simulink model "MultiMicrogrid"  (R2022b)
settings: Solver=ode45  StartTime=0.0  StopTime=1000  RelTol=1e-3  AbsTol=1e-5
values from neighbouring files (symbols this model uses):
  a_hidden_weights1 = zeros(n,h)    [Weights.m]
  a_hidden_weights2 = zeros(n,h)    [Weights.m]
  a_hidden_weights3 = zeros(n,h)    [Weights.m]
  a_input_weights1 = zeros(h,m)    [Weights.m]
  a_input_weights2 = zeros(h,m)    [Weights.m]
  a_input_weights3 = zeros(h,m)    [Weights.m]
  c_hidden_weights11 = zeros(100,1000)    [Training.m]
  c_hidden_weights12 = -1+(1+1)*rand(1,100,'single')    [Training.m]
  c_hidden_weights21 = zeros(100,1000)    [Training.m]
  c_hidden_weights22 = -1+(1+1)*rand(1,100,'single')    [Training.m]
  c_hidden_weights31 = zeros(100,1000)    [Training.m]
  c_hidden_weights32 = -1+(1+1)*rand(1,100,'single')    [Training.m]
  c_hidden_weights_a1 = -1+(1+1)*rand(1,100,'single')    [Training.m]
  c_hidden_weights_a2 = -1+(1+1)*rand(1,100,'single')    [Training.m]
  c_hidden_weights_a3 = -1+(1+1)*rand(1,100,'single')    [Training.m]
  c_input_weights1 = zeros(1000,m)    [Training.m]
  c_input_weights2 = zeros(1000,m)    [Training.m]
  c_input_weights3 = zeros(1000,m)    [Training.m]
  c_input_weights_a1 = zeros(100,n)    [Training.m]
  c_input_weights_a2 = zeros(100,n)    [Training.m]
  c_input_weights_a3 = zeros(100,n)    [Training.m]
libraries: simulink x27, fuzblock x3, mpclib x3, slpidlib x3
(part 1 of 2)
settings Model: Creator=Vjatšeslav Škiparev  LastModifiedBy=Vjatšeslav Škiparev
settings DataIOCC: SaveState=on  StateSaveName=xout2  TimeSaveName=time  LoggingIntervals=[0, 1000]
settings DebuggingCC: UnconnectedInputMsg=warning  UnconnectedOutputMsg=warning  UnconnectedLineMsg=warning
settings HardwareCC: ProdBitPerLong=64  ProdHWDeviceType=Intel->x86-64 (Linux 64)
settings ModelReferenceCC: EnableRefExpFcnMdlSchedulingChecks=on
settings RTWCC: DLArmComputeVersion=19.05

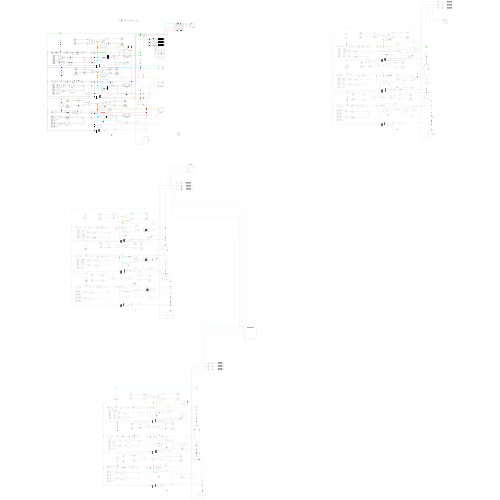
[thumbnail: Simulink's stored preview of the top-level diagram]
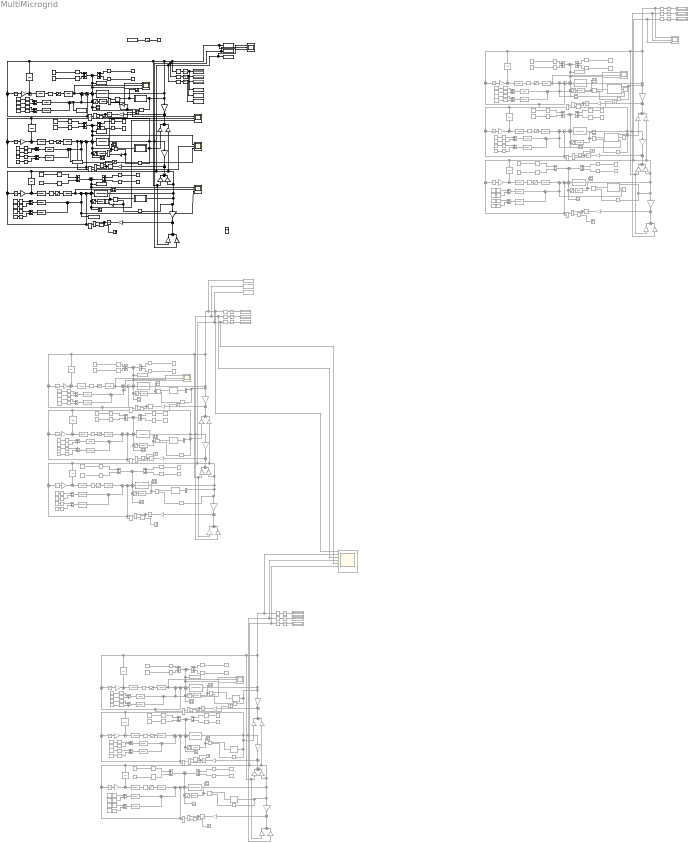
== system MultiMicrogrid ==
  Abs : Abs  SaturateOnIntegerOverflow=off
  Abs1 : Abs  SaturateOnIntegerOverflow=off
  Abs{3..11} (9 alike) : Abs  Commented=on  SaturateOnIntegerOverflow=off
  Abs2 : Abs  SaturateOnIntegerOverflow=off
  Agent 1 : Subsystem
  Agent 2 : Subsystem
  Agent 3 : Subsystem
  Constant : Constant  Value=0.1
  Constant1 : Constant  Value=-0.1
  Constant2 : Constant  SampleTime=1
  Constant3 : Constant  Commented=on  Value=0
  Constant4 : Constant  Commented=on  Value=0
  Constant5 : Constant  Commented=on  Value=0
  Deadband : DeadZone  LowerValue=-0.12  UpperValue=0.12
  Derivative1 : Derivative
  Derivative{4..12} (9 alike) : Derivative  Commented=on
  Derivative2 : Derivative
  Derivative3 : Derivative
  Display : Display
  Display1 : Display
  Display{3..11} (9 alike) : Display  Commented=on
  Display2 : Display
  First Order Hold{1..24} (24 alike) : FirstOrderHold  ErrorTolerance=inf
  First Order Hold{25..96} (72 alike) : FirstOrderHold  Commented=on  ErrorTolerance=inf
  Frequency : Scope  Commented=on  NumInputPorts=8
  Fuzzy Logic Controller1 : fuzblock/Fuzzy Logic  Controller  Commented=on  FIS='test.fis'  OutputSampleNumber=101  DataType=double  FuzzifiedInputs=off  RuleFiringStrengths=off  RuleOutputs=off  AggregatedOutputs=off  SimulateUsing=Interpreted execution  OutOfRangeInputValueMessage=warning  NoRuleFiredMessage=warning  EmptyOutputFuzzySetMessage=warning
  Fuzzy Logic Controller2 : fuzblock/Fuzzy Logic  Controller  Commented=on  FIS='test.fis'  OutputSampleNumber=101  DataType=double  FuzzifiedInputs=off  RuleFiringStrengths=off  RuleOutputs=off  AggregatedOutputs=off  SimulateUsing=Interpreted execution  OutOfRangeInputValueMessage=warning  NoRuleFiredMessage=warning  EmptyOutputFuzzySetMessage=warning
  Fuzzy Logic Controller3 : fuzblock/Fuzzy Logic  Controller  Commented=on  FIS='test.fis'  OutputSampleNumber=101  DataType=double  FuzzifiedInputs=off  RuleFiringStrengths=off  RuleOutputs=off  AggregatedOutputs=off  SimulateUsing=Interpreted execution  OutOfRangeInputValueMessage=warning  NoRuleFiredMessage=warning  EmptyOutputFuzzySetMessage=warning
  GRC : DeadZone  LowerValue=-0.12  UpperValue=0.12
  GRC{1,3..10} (9 alike) : DeadZone  Commented=on  LowerValue=-0.12  UpperValue=0.12
  GRC11 : Saturate  UpperLimit=0.4  LowerLimit=0
  GRC2 : DeadZone  LowerValue=-0.12  UpperValue=0.12
  Gain : Gain  Gain=0.25
  Gain1 : Gain  Gain=0.2
  Gain10 : Gain  Gain=3.14*2
  Gain11 : Gain  Gain=3.14*2
  Gain12 : Gain  Gain=0.2+0.25
  Gain13 : Gain  Gain=0.2+0.12
  Gain14 : Gain  Gain=0.25+0.25
  Gain15 : Gain  Gain=-0.6
  Gain16 : Gain  Gain=-0.6
  Gain17 : Gain  Gain=-0.6
  Gain{18,25,31,33,43,45,49,60,62} (9 alike) : Gain  Commented=on  Gain=0.25
  Gain{19,26,32,44,50,61} (6 alike) : Gain  Commented=on  Gain=0.2
  Gain2 : Gain  Gain=-0.40
  Gain{20..21,27,35..36,47,51,53,64} (9 alike) : Gain  Commented=on  Gain=3.14*2
  Gain22 : Gain  Commented=on  Gain=0.2+0.25
  Gain23 : Gain  Commented=on  Gain=0.2+0.12
  Gain24 : Gain  Commented=on  Gain=0.25+0.25
  Gain28 : Gain  Commented=on  Gain=-0.40
  Gain29 : Gain  Commented=on  Gain=-0.25
  Gain3 : Gain  Gain=-0.25
  Gain30 : Gain  Commented=on  Gain=0.12
  Gain34 : Gain  Commented=on  Gain=-0.35
  Gain37 : Gain  Commented=on  Gain=0.2+0.25
  Gain38 : Gain  Commented=on  Gain=0.2+0.12
  Gain39 : Gain  Commented=on  Gain=0.25+0.25
  Gain4 : Gain  Gain=0.12
  Gain40 : Gain  Commented=on  Gain=-0.40
  Gain41 : Gain  Commented=on  Gain=-0.25
  Gain42 : Gain  Commented=on  Gain=0.12
  Gain46 : Gain  Commented=on  Gain=-0.35
  Gain5 : Gain  Gain=0.25
  Gain54 : Gain  Commented=on  Gain=0.2+0.25
  Gain55 : Gain  Commented=on  Gain=0.2+0.12
  Gain56 : Gain  Commented=on  Gain=0.25+0.25
  Gain57 : Gain  Commented=on  Gain=-0.40
  Gain58 : Gain  Commented=on  Gain=-0.25
  Gain59 : Gain  Commented=on  Gain=0.12
  Gain6 : Gain  Gain=0.2
  Gain63 : Gain  Commented=on  Gain=-0.35
  Gain7 : Gain  Gain=0.25
  Gain8 : Gain  Gain=-0.35
  Gain9 : Gain  Gain=3.14*2
  Industrial Loads1 : UniformRandomNumber  Minimum=-0.01  Maximum=0.01  SampleTime=1
  Industrial Loads{9..10,13,18..19,24} (6 alike) : UniformRandomNumber  Commented=on  Minimum=-0.03  Maximum=0.03  SampleTime=5
  Industrial Loads{11..12,14..15,20..21} (6 alike) : UniformRandomNumber  Commented=on  Minimum=-0.01  Maximum=0.01  SampleTime=2
  Industrial Loads16 : UniformRandomNumber  Commented=on  Minimum=-0.01  Maximum=0.01  SampleTime=1
  Industrial Loads17 : UniformRandomNumber  Commented=on  Minimum=-0.05  Maximum=0.05  SampleTime=2
  Industrial Loads2 : UniformRandomNumber  Minimum=-0.05  Maximum=0.05  SampleTime=2
  Industrial Loads22 : UniformRandomNumber  Commented=on  Minimum=-0.01  Maximum=0.01  SampleTime=1
  Industrial Loads23 : UniformRandomNumber  Commented=on  Minimum=-0.05  Maximum=0.05  SampleTime=2
  Industrial Loads3 : UniformRandomNumber  Minimum=-0.03  Maximum=0.03  SampleTime=5
  Industrial Loads4 : UniformRandomNumber  Minimum=-0.03  Maximum=0.03  SampleTime=5
  Industrial Loads5 : UniformRandomNumber  Minimum=-0.01  Maximum=0.01  SampleTime=2
  Industrial Loads6 : UniformRandomNumber  Minimum=-0.01  Maximum=0.01  SampleTime=2
  Industrial Loads7 : UniformRandomNumber  Commented=on  Minimum=-0.01  Maximum=0.01  SampleTime=1
  Industrial Loads8 : UniformRandomNumber  Commented=on  Minimum=-0.05  Maximum=0.05  SampleTime=2
  Integrator{,1..9} (10 alike) : Integrator
  Integrator{10..36} (27 alike) : Integrator  Commented=on
  Limiter1 : Saturate  Commented=on  UpperLimit=0.4  LowerLimit=0
  Limiter10 : Saturate  Commented=on  LowerLimit=0
  Limiter11 : Saturate  Commented=on  UpperLimit=0.3  LowerLimit=0
  Limiter2 : Saturate  LowerLimit=0
  Limiter3 : Saturate  UpperLimit=0.3  LowerLimit=0
  Limiter4 : Saturate  Commented=on  UpperLimit=0.4  LowerLimit=0
  Limiter5 : Saturate  Commented=on  LowerLimit=0
  Limiter6 : Saturate  Commented=on  UpperLimit=0.3  LowerLimit=0
  Limiter7 : Saturate  Commented=on  LowerLimit=0
  Limiter8 : Saturate  Commented=on  UpperLimit=0.3  LowerLimit=0
  Limiter9 : Saturate  Commented=on  UpperLimit=0.4  LowerLimit=0
  MPC Controller : mpclib/MPC Controller  Commented=on  SCDEnableBlockLinearizationSpecification=on  is_multiple=0  enable_value=0  return_u0=off  updateMPCinCallerWorkspace=on  md_inport=on  mv_inport=off  uref_inport=off  return_cost=off  return_mvseq=off  return_qpstatus=off  return_xseq=off  return_state=off  return_ovseq=off  state_inport=off  umin_inport=off  umax_inport=off  ymin_inport=off  ymax_inport=off  cc_inport=off  ywt_inport=off  uwt_inport=off  duwt_inport=off  rhoeps_inport=off  pm_inport=off  MaximumP=10  HorizonChoice=FixedHorizon  n_ts=1  n_p=10  n_mv=1  n_md=1  n_ud=0  n_mo=1  n_uo=0  BlockDataType=double  SampleTimeInherited=off  switch_inport=off
  MPC Controller1 : mpclib/MPC Controller  Commented=on  SCDEnableBlockLinearizationSpecification=on  is_multiple=0  enable_value=0  return_u0=off  updateMPCinCallerWorkspace=on  md_inport=on  mv_inport=off  uref_inport=off  return_cost=off  return_mvseq=off  return_qpstatus=off  return_xseq=off  return_state=off  return_ovseq=off  state_inport=off  umin_inport=off  umax_inport=off  ymin_inport=off  ymax_inport=off  cc_inport=off  ywt_inport=off  uwt_inport=off  duwt_inport=off  rhoeps_inport=off  pm_inport=off  MaximumP=10  HorizonChoice=FixedHorizon  n_ts=1  n_p=10  n_mv=1  n_md=1  n_ud=0  n_mo=1  n_uo=0  BlockDataType=double  SampleTimeInherited=off  switch_inport=off
  MPC Controller2 : mpclib/MPC Controller  Commented=on  SCDEnableBlockLinearizationSpecification=on  mpcobj=mpc1  is_multiple=0  enable_value=0  return_u0=off  updateMPCinCallerWorkspace=on  md_inport=on  mv_inport=off  uref_inport=off  return_cost=off  return_mvseq=off  return_qpstatus=off  return_xseq=off  return_state=off  return_ovseq=off  state_inport=off  umin_inport=off  umax_inport=off  ymin_inport=off  ymax_inport=off  cc_inport=off  ywt_inport=off  uwt_inport=off  duwt_inport=off  rhoeps_inport=off  pm_inport=off  MaximumP=10  HorizonChoice=FixedHorizon  n_ts=1  n_p=10  n_mv=1  n_md=1  n_ud=0  n_mo=1  n_uo=0  BlockDataType=double  SampleTimeInherited=off  switch_inport=off
  Manual Variant Source{6..11} (6 alike) : simulink/Signal Routing/Manual Variant Source  NumChoices=2  LabelModeActiveChoice=V_2
  Manual Variant Source{2,12..14,16..19,22,24..28} (14 alike) : simulink/Signal Routing/Manual Variant Source  Commented=on  NumChoices=2  LabelModeActiveChoice=V_2
  Manual Variant Source{15,20..21,23} (4 alike) : simulink/Signal Routing/Manual Variant Source  Commented=on  NumChoices=2  LabelModeActiveChoice=V_1
  Manual Variant Source3 : simulink/Signal Routing/Manual Variant Source  NumChoices=2  LabelModeActiveChoice=V_1
  Manual Variant Source4 : simulink/Signal Routing/Manual Variant Source  NumChoices=2  LabelModeActiveChoice=V_1
  Manual Variant Source5 : simulink/Signal Routing/Manual Variant Source  NumChoices=2  LabelModeActiveChoice=V_1
  Mux1 : Mux  Commented=on  Inputs=2
  Mux2 : Mux  Commented=on  Inputs=2
  Mux3 : Mux  Commented=on  Inputs=2
  PID Controller1 : slpidlib/PID Controller  Commented=on  Controller=PID  Form=Parallel  TimeDomain=Continuous-time  UseExternalTs=off  SampleTime=-1  IntegratorMethod=Forward Euler  FilterMethod=Forward Euler  ControllerParametersSource=internal  P=7.5  I=2.5  UseKiTs=off  D=0.75  N=100  UseFilter=on  TunerSelectOption=Transfer Function Based (PID Tuner App)  InitialConditionSource=internal  InitialConditionForIntegrator=0  InitialConditionForFilter=0  DifferentiatorICPrevScaledInput=0  ExternalReset=none  TrackingMode=off  Kt=1  LimitOutput=off  SatLimitsSource=internal  UpperSaturationLimit=inf  LowerSaturationLimit=0  LinearizeAsGain=on  AntiWindupMode=none  Kb=1  LimitIntegrator=off  UpperIntegratorSaturationLimit=inf  LowerIntegratorSaturationLimit=-inf  POutMin=[]  POutMax=[]  IOutMin=[]  IOutMax=[]  DOutMin=[]  DOutMax=[]  NOutMin=[]  NOutMax=[]  SumOutMin=[]  SumOutMax=[]  SaturationOutMin=[]  SaturationOutMax=[]  PParamMin=[]  PParamMax=[]  IParamMin=[]  IParamMax=[]  DParamMin=[]  DParamMax=[]  NParamMin=[]  NParamMax=[]  KbParamMin=[]  KbParamMax=[]  KtParamMin=[]  KtParamMax=[]  KbOutMin=[]  KbOutMax=[]  KtOutMin=[]  KtOutMax=[]  IntegratorOutMin=[]  IntegratorOutMax=[]  FilterOutMin=[]  FilterOutMax=[]  SumI1OutMin=[]  SumI1OutMax=[]  SumI2OutMin=[]  SumI2OutMax=[]  SumI3OutMin=[]  SumI3OutMax=[]  SumI4OutMin=[]  SumI4OutMax=[]  SumDOutMin=[]  SumDOutMax=[]  DifferentiatorOutMin=[]  DifferentiatorOutMax=[]  FilterDiffOutCoefMin=[]  FilterDiffOutCoefMax=[]  ReciprocalOutMin=[]  ReciprocalOutMax=[]  SumDenOutMin=[]  SumDenOutMax=[]  SumNumOutMin=[]  SumNumOutMax=[]  DivideOutMin=[]  DivideOutMax=[]  UdiffTsProdOutMin=[]  UdiffTsProdOutMax=[]  NTsProdOutMin=[]  NTsProdOutMax=[]  UintegralTsProdOutMin=[]  UintegralTsProdOutMax=[]  UngainTsProdOutMin=[]  UngainTsProdOutMax=[]  ClampingZeroOutDataTypeStr=Inherit: Inherit via back propagation  ClampingZeroOutMin=[]  ClampingZeroOutMax=[]  FilterDenConstantOutDataTypeStr=Inherit: Inherit via back propagation  FilterDenConstantOutMin=[]  FilterDenConstantOutMax=[]  PCopyOutDataTypeStr=Inherit: Inherit via back propagation  PCopyOutMin=[]  PCopyOutMax=[]  NCopyOutDataTypeStr=Inherit: Inherit via back propagation  NCopyOutMin=[]  NCopyOutMax=[]  IntegratorContinuousStateAttributes=''  IntegratorStateMustResolveToSignalObject=off  IntegratorRTWStateStorageClass=Auto  FilterContinuousStateAttributes=''  FilterStateMustResolveToSignalObject=off  FilterRTWStateStorageClass=Auto  ParallelPVariant=InternalParameters  IdealPVariant=Disabled  IVariant=InternalParameters  DVariant=InternalParameters  IntegratorVariant=Continuous  SatVariant=Disabled  AWVariant=Passthrough  PCopyVariant=Disabled  TRVariant=Disabled  FdbkBlocksVariant=Forward  IdealPFdbkVariant=Disabled  SatFdbkVariant=Disabled  DerivativeFilterVariant=ContFilter  NVariant=InternalParameters  NCopyVariant=Disabled  FilterICVariant=InternalICsFilter  IntegratorICVariant=InternalICs  ExternalResetVariant=Disabled  TRSumVariant=Passthrough  SumFdbkVariant=Disabled  SumVariant=Sum_PID  TsampFilterVariant=InternalTs  TsampNgainVariant=Passthrough  TsampIntegralVariant=Passthrough  ExternalSaturationOutDataTypeStr=Inherit: Same as second input
  PID Controller2 : slpidlib/PID Controller  Commented=on  Controller=PID  Form=Parallel  TimeDomain=Continuous-time  UseExternalTs=off  SampleTime=-1  IntegratorMethod=Forward Euler  FilterMethod=Forward Euler  ControllerParametersSource=internal  P=4.75  I=1.25  UseKiTs=off  D=0.5  N=100  UseFilter=on  TunerSelectOption=Transfer Function Based (PID Tuner App)  InitialConditionSource=internal  InitialConditionForIntegrator=0  InitialConditionForFilter=0  DifferentiatorICPrevScaledInput=0  ExternalReset=none  TrackingMode=off  Kt=1  LimitOutput=off  SatLimitsSource=internal  UpperSaturationLimit=inf  LowerSaturationLimit=-inf  LinearizeAsGain=on  AntiWindupMode=back-calculation  Kb=1  LimitIntegrator=off  UpperIntegratorSaturationLimit=inf  LowerIntegratorSaturationLimit=-inf  POutMin=[]  POutMax=[]  IOutMin=[]  IOutMax=[]  DOutMin=[]  DOutMax=[]  NOutMin=[]  NOutMax=[]  SumOutMin=[]  SumOutMax=[]  SaturationOutMin=[]  SaturationOutMax=[]  PParamMin=[]  PParamMax=[]  IParamMin=[]  IParamMax=[]  DParamMin=[]  DParamMax=[]  NParamMin=[]  NParamMax=[]  KbParamMin=[]  KbParamMax=[]  KtParamMin=[]  KtParamMax=[]  KbOutMin=[]  KbOutMax=[]  KtOutMin=[]  KtOutMax=[]  IntegratorOutMin=[]  IntegratorOutMax=[]  FilterOutMin=[]  FilterOutMax=[]  SumI1OutMin=[]  SumI1OutMax=[]  SumI2OutMin=[]  SumI2OutMax=[]  SumI3OutMin=[]  SumI3OutMax=[]  SumI4OutMin=[]  SumI4OutMax=[]  SumDOutMin=[]  SumDOutMax=[]  DifferentiatorOutMin=[]  DifferentiatorOutMax=[]  FilterDiffOutCoefMin=[]  FilterDiffOutCoefMax=[]  ReciprocalOutMin=[]  ReciprocalOutMax=[]  SumDenOutMin=[]  SumDenOutMax=[]  SumNumOutMin=[]  SumNumOutMax=[]  DivideOutMin=[]  DivideOutMax=[]  UdiffTsProdOutMin=[]  UdiffTsProdOutMax=[]  NTsProdOutMin=[]  NTsProdOutMax=[]  UintegralTsProdOutMin=[]  UintegralTsProdOutMax=[]  UngainTsProdOutMin=[]  UngainTsProdOutMax=[]  ClampingZeroOutDataTypeStr=Inherit: Inherit via back propagation  ClampingZeroOutMin=[]  ClampingZeroOutMax=[]  FilterDenConstantOutDataTypeStr=Inherit: Inherit via back propagation  FilterDenConstantOutMin=[]  FilterDenConstantOutMax=[]  PCopyOutDataTypeStr=Inherit: Inherit via back propagation  PCopyOutMin=[]  PCopyOutMax=[]  NCopyOutDataTypeStr=Inherit: Inherit via back propagation  NCopyOutMin=[]  NCopyOutMax=[]  IntegratorContinuousStateAttributes=''  IntegratorStateMustResolveToSignalObject=off  IntegratorRTWStateStorageClass=Auto  FilterContinuousStateAttributes=''  FilterStateMustResolveToSignalObject=off  FilterRTWStateStorageClass=Auto  ParallelPVariant=InternalParameters  IdealPVariant=Disabled  IVariant=InternalParameters  DVariant=InternalParameters  IntegratorVariant=Continuous  SatVariant=Disabled  AWVariant=Passthrough  PCopyVariant=Disabled  TRVariant=Disabled  FdbkBlocksVariant=Forward  IdealPFdbkVariant=Disabled  SatFdbkVariant=Disabled  DerivativeFilterVariant=ContFilter  NVariant=InternalParameters  NCopyVariant=Disabled  FilterICVariant=InternalICsFilter  IntegratorICVariant=InternalICs  ExternalResetVariant=Disabled  TRSumVariant=Passthrough  SumFdbkVariant=Disabled  SumVariant=Sum_PID  TsampFilterVariant=InternalTs  TsampNgainVariant=Passthrough  TsampIntegralVariant=Passthrough  ExternalSaturationOutDataTypeStr=Inherit: Same as second input
  PID Controller3 : slpidlib/PID Controller  Commented=on  Controller=PID  Form=Parallel  TimeDomain=Continuous-time  UseExternalTs=off  SampleTime=-1  IntegratorMethod=Forward Euler  FilterMethod=Forward Euler  ControllerParametersSource=internal  P=4.5  I=1.75  UseKiTs=off  D=0.2  N=100  UseFilter=on  TunerSelectOption=Transfer Function Based (PID Tuner App)  InitialConditionSource=internal  InitialConditionForIntegrator=0  InitialConditionForFilter=0  DifferentiatorICPrevScaledInput=0  ExternalReset=none  TrackingMode=off  Kt=1  LimitOutput=off  SatLimitsSource=internal  UpperSaturationLimit=inf  LowerSaturationLimit=0  LinearizeAsGain=on  AntiWindupMode=none  Kb=1  LimitIntegrator=off  UpperIntegratorSaturationLimit=inf  LowerIntegratorSaturationLimit=-inf  POutMin=[]  POutMax=[]  IOutMin=[]  IOutMax=[]  DOutMin=[]  DOutMax=[]  NOutMin=[]  NOutMax=[]  SumOutMin=[]  SumOutMax=[]  SaturationOutMin=[]  SaturationOutMax=[]  PParamMin=[]  PParamMax=[]  IParamMin=[]  IParamMax=[]  DParamMin=[]  DParamMax=[]  NParamMin=[]  NParamMax=[]  KbParamMin=[]  KbParamMax=[]  KtParamMin=[]  KtParamMax=[]  KbOutMin=[]  KbOutMax=[]  KtOutMin=[]  KtOutMax=[]  IntegratorOutMin=[]  IntegratorOutMax=[]  FilterOutMin=[]  FilterOutMax=[]  SumI1OutMin=[]  SumI1OutMax=[]  SumI2OutMin=[]  SumI2OutMax=[]  SumI3OutMin=[]  SumI3OutMax=[]  SumI4OutMin=[]  SumI4OutMax=[]  SumDOutMin=[]  SumDOutMax=[]  DifferentiatorOutMin=[]  DifferentiatorOutMax=[]  FilterDiffOutCoefMin=[]  FilterDiffOutCoefMax=[]  ReciprocalOutMin=[]  ReciprocalOutMax=[]  SumDenOutMin=[]  SumDenOutMax=[]  SumNumOutMin=[]  SumNumOutMax=[]  DivideOutMin=[]  DivideOutMax=[]  UdiffTsProdOutMin=[]  UdiffTsProdOutMax=[]  NTsProdOutMin=[]  NTsProdOutMax=[]  UintegralTsProdOutMin=[]  UintegralTsProdOutMax=[]  UngainTsProdOutMin=[]  UngainTsProdOutMax=[]  ClampingZeroOutDataTypeStr=Inherit: Inherit via back propagation  ClampingZeroOutMin=[]  ClampingZeroOutMax=[]  FilterDenConstantOutDataTypeStr=Inherit: Inherit via back propagation  FilterDenConstantOutMin=[]  FilterDenConstantOutMax=[]  PCopyOutDataTypeStr=Inherit: Inherit via back propagation  PCopyOutMin=[]  PCopyOutMax=[]  NCopyOutDataTypeStr=Inherit: Inherit via back propagation  NCopyOutMin=[]  NCopyOutMax=[]  IntegratorContinuousStateAttributes=''  IntegratorStateMustResolveToSignalObject=off  IntegratorRTWStateStorageClass=Auto  FilterContinuousStateAttributes=''  FilterStateMustResolveToSignalObject=off  FilterRTWStateStorageClass=Auto  ParallelPVariant=InternalParameters  IdealPVariant=Disabled  IVariant=InternalParameters  DVariant=InternalParameters  IntegratorVariant=Continuous  SatVariant=Disabled  AWVariant=Passthrough  PCopyVariant=Disabled  TRVariant=Disabled  FdbkBlocksVariant=Forward  IdealPFdbkVariant=Disabled  SatFdbkVariant=Disabled  DerivativeFilterVariant=ContFilter  NVariant=InternalParameters  NCopyVariant=Disabled  FilterICVariant=InternalICsFilter  IntegratorICVariant=InternalICs  ExternalResetVariant=Disabled  TRSumVariant=Passthrough  SumFdbkVariant=Disabled  SumVariant=Sum_PID  TsampFilterVariant=InternalTs  TsampNgainVariant=Passthrough  TsampIntegralVariant=Passthrough  ExternalSaturationOutDataTypeStr=Inherit: Same as second input
  PowerPlant1 : Scope  NumInputPorts=3
  PowerPlant2 : Scope  NumInputPorts=3
  PowerPlant3 : Scope  NumInputPorts=3
  PowerPlant{4..7} (4 alike) : Scope  Commented=on  NumInputPorts=3
  Product{,1..5} (6 alike) : Product
  Product{6..23} (18 alike) : Product  Commented=on
  Reward1 : ToWorkspace  VariableName=axis  SampleTime=1
      settings: Save2DSignal=2-D array (concatenate along first dimension)
  Saturation : Saturate  UpperLimit=0.25  LowerLimit=-0.25
  Saturation1 : Saturate  UpperLimit=0.1  LowerLimit=-0.1
  Saturation10 : Saturate  Commented=on  UpperLimit=0.1  LowerLimit=-0.1
  Saturation11 : Saturate  Commented=on  UpperLimit=0.2  LowerLimit=-0.2
  Saturation2 : Saturate  UpperLimit=0.2  LowerLimit=-0.2
  Saturation3 : Saturate  Commented=on  UpperLimit=0.25  LowerLimit=-0.25
  Saturation4 : Saturate  Commented=on  UpperLimit=0.1  LowerLimit=-0.1
  Saturation5 : Saturate  Commented=on  UpperLimit=0.2  LowerLimit=-0.2
  Saturation6 : Saturate  Commented=on  UpperLimit=0.25  LowerLimit=-0.25
  Saturation7 : Saturate  Commented=on  UpperLimit=0.1  LowerLimit=-0.1
  Saturation8 : Saturate  Commented=on  UpperLimit=0.2  LowerLimit=-0.2
  Saturation9 : Saturate  Commented=on  UpperLimit=0.25  LowerLimit=-0.25
  Scope{,1..5} (6 alike) : Scope
  Scope{6..23} (18 alike) : Scope  Commented=on
  Solar1 : TransferFcn  Denominator=[1.5 1]
  Solar10 : TransferFcn  Commented=on  Denominator=[1.5 1]
  Solar11 : TransferFcn  Commented=on  Denominator=[1.3 1]
  Solar12 : TransferFcn  Commented=on  Denominator=[1.75 1]
  Solar2 : TransferFcn  Denominator=[1.3 1]
  Solar3 : TransferFcn  Denominator=[1.75 1]
  Solar4 : TransferFcn  Commented=on  Denominator=[1.5 1]
  Solar5 : TransferFcn  Commented=on  Denominator=[1.3 1]
  Solar6 : TransferFcn  Commented=on  Denominator=[1.75 1]
  Solar7 : TransferFcn  Commented=on  Denominator=[1.5 1]
  Solar8 : TransferFcn  Commented=on  Denominator=[1.3 1]
  Solar9 : TransferFcn  Commented=on  Denominator=[1.75 1]
  Step : Step  Time=750  Before=1  After=0  SampleTime=0
  Step1 : Step  Time=250  Before=1  After=0  SampleTime=0
  Step10 : Step  Commented=on  Time=250  Before=1  After=0  SampleTime=0
  Step11 : Step  Commented=on  Time=500  Before=1  After=0  SampleTime=0
  Step2 : Step  Time=500  Before=1  After=0  SampleTime=0
  Step3 : Step  Commented=on  Time=750  Before=1  After=0  SampleTime=0
  Step4 : Step  Commented=on  Time=250  Before=1  After=0  SampleTime=0
  Step5 : Step  Commented=on  Time=500  Before=1  After=0  SampleTime=0
  Step6 : Step  Commented=on  Time=750  Before=1  After=0  SampleTime=0
  Step7 : Step  Commented=on  Time=250  Before=1  After=0  SampleTime=0
  Step8 : Step  Commented=on  Time=500  Before=1  After=0  SampleTime=0
  Step9 : Step  Commented=on  Time=750  Before=1  After=0  SampleTime=0
  Sum : Sum  Inputs=-++
  Sum1 : Sum  Inputs=-++
  Sum{9..11,15..17,24..38} (21 alike) : Sum
  Sum{41..42,46..48,56..61,63..71,77,80..81,85..87,95..100,102..110,116..117,119..127,133,136..137,141..143,151..155} (63 alike) : Sum  Commented=on
  Sum{62,72..73,101,111..112,118,128..129} (9 alike) : Sum  Commented=on  Inputs=-+|
  Sum{74..76,113..115,130..132} (9 alike) : Sum  Commented=on  Inputs=+-
  Sum12 : Sum  Inputs=|+-
  Sum13 : Sum  Inputs=|+-
  Sum{39..40,51,78..79,90,134..135,146} (9 alike) : Sum  Commented=on  Inputs=-++
  Sum{43..45,82..84,138..140} (9 alike) : Sum  Commented=on  Inputs=|+-
  Sum14 : Sum  Inputs=|+-
  Sum{49..50,52..55,88..89,91..94,144..145,147..150} (18 alike) : Sum  Commented=on  Inputs=|++
  Sum{18..23} (6 alike) : Sum  Inputs=|++
  Sum2 : Sum  Inputs=-++
  Sum3 : Sum  Inputs=-+|
  Sum4 : Sum  Inputs=-+|
  Sum5 : Sum  Inputs=-+|
  Sum6 : Sum  Inputs=+-
  Sum7 : Sum  Inputs=+-
  Sum8 : Sum  Inputs=+-
  To Workspace : ToWorkspace  VariableName=frequency1  SampleTime=1
  To Workspace1 : ToWorkspace  VariableName=frequency2  SampleTime=1
  To Workspace10 : ToWorkspace  VariableName=IAE2  SampleTime=1
  To Workspace11 : ToWorkspace  VariableName=IAE1  SampleTime=1
  To Workspace12 : ToWorkspace  Commented=on  VariableName=Load  SampleTime=1
  To Workspace13 : ToWorkspace  Commented=on  VariableName=Load4  SampleTime=1
  To Workspace14 : ToWorkspace  Commented=on  VariableName=Load5  SampleTime=1
  To Workspace15 : ToWorkspace  Commented=on  VariableName=frequency  SampleTime=1
  To Workspace16 : ToWorkspace  Commented=on  VariableName=frequency4  SampleTime=1
  To Workspace17 : ToWorkspace  Commented=on  VariableName=frequency5  SampleTime=1
  To Workspace2 : ToWorkspace  VariableName=frequency3  SampleTime=1
  To Workspace3 : ToWorkspace  VariableName=Load1  SampleTime=1
  To Workspace4 : ToWorkspace  VariableName=Load2  SampleTime=1
  To Workspace5 : ToWorkspace  VariableName=Load3  SampleTime=1
  To Workspace6 : ToWorkspace  VariableName=RES2  SampleTime=1
  To Workspace7 : ToWorkspace  VariableName=RES1  SampleTime=1
  To Workspace8 : ToWorkspace  VariableName=RES3  SampleTime=1
  To Workspace9 : ToWorkspace  VariableName=IAE3  SampleTime=1
  Transfer Fcn : TransferFcn  Denominator=[0.1 1]
  Transfer Fcn1 : TransferFcn  Denominator=[0.4 1]
  Transfer Fcn10 : TransferFcn  Denominator=[3.0]
  Transfer Fcn11 : TransferFcn  Denominator=[2.4]
  Transfer Fcn12 : TransferFcn  Denominator=[10 1]
  Transfer Fcn13 : TransferFcn  Denominator=[8.5 1]
  Transfer Fcn14 : TransferFcn  Denominator=[12 1]
  Transfer Fcn15 : TransferFcn  Commented=on  Denominator=[0.1 1]
  Transfer Fcn16 : TransferFcn  Commented=on  Denominator=[0.4 1]
  Transfer Fcn17 : TransferFcn  Commented=on  Denominator=[3.0]
  Transfer Fcn18 : TransferFcn  Commented=on  Denominator=[2.4]
  Transfer Fcn19 : TransferFcn  Commented=on  Denominator=[10 1]
  Transfer Fcn2 : TransferFcn  Denominator=[0.12 1]
  Transfer Fcn20 : TransferFcn  Commented=on  Denominator=[8.5 1]
  Transfer Fcn21 : TransferFcn  Commented=on  Denominator=[12 1]
  Transfer Fcn22 : TransferFcn  Commented=on  Denominator=[0.12 1]
  Transfer Fcn23 : TransferFcn  Commented=on  Denominator=[0.45 1]
  Transfer Fcn24 : TransferFcn  Commented=on  Denominator=[0.15 1]
  Transfer Fcn25 : TransferFcn  Commented=on  Denominator=[0.35 1]
  Transfer Fcn26 : TransferFcn  Commented=on  Denominator=[2*0.083 0.015]
  Transfer Fcn27 : TransferFcn  Commented=on  Denominator=[2*0.1 0.017]
  Transfer Fcn28 : TransferFcn  Commented=on  Denominator=[2*0.0623 0.014]
  Transfer Fcn29 : TransferFcn  Commented=on  Denominator=[2.73]
  Transfer Fcn3 : TransferFcn  Denominator=[0.45 1]
  Transfer Fcn30 : TransferFcn  Commented=on  Denominator=[0.1 1]
  Transfer Fcn31 : TransferFcn  Commented=on  Denominator=[0.4 1]
  Transfer Fcn32 : TransferFcn  Commented=on  Denominator=[3.0]
  Transfer Fcn33 : TransferFcn  Commented=on  Denominator=[2.4]
  Transfer Fcn34 : TransferFcn  Commented=on  Denominator=[10 1]
  Transfer Fcn35 : TransferFcn  Commented=on  Denominator=[8.5 1]
  Transfer Fcn36 : TransferFcn  Commented=on  Denominator=[12 1]
  Transfer Fcn37 : TransferFcn  Commented=on  Denominator=[0.12 1]
  Transfer Fcn38 : TransferFcn  Commented=on  Denominator=[0.45 1]
  Transfer Fcn39 : TransferFcn  Commented=on  Denominator=[0.15 1]
  Transfer Fcn4 : TransferFcn  Denominator=[0.15 1]
  Transfer Fcn40 : TransferFcn  Commented=on  Denominator=[0.35 1]
  Transfer Fcn41 : TransferFcn  Commented=on  Denominator=[2*0.083 0.015]
  Transfer Fcn42 : TransferFcn  Commented=on  Denominator=[2*0.1 0.017]
  Transfer Fcn43 : TransferFcn  Commented=on  Denominator=[2*0.0623 0.014]
  Transfer Fcn44 : TransferFcn  Commented=on  Denominator=[2.73]
  Transfer Fcn45 : TransferFcn  Commented=on  Denominator=[0.1 1]
  Transfer Fcn46 : TransferFcn  Commented=on  Denominator=[0.4 1]
  Transfer Fcn47 : TransferFcn  Commented=on  Denominator=[3.0]
  Transfer Fcn48 : TransferFcn  Commented=on  Denominator=[2.4]
  Transfer Fcn49 : TransferFcn  Commented=on  Denominator=[10 1]
  Transfer Fcn5 : TransferFcn  Denominator=[0.35 1]
  Transfer Fcn50 : TransferFcn  Commented=on  Denominator=[8.5 1]
  Transfer Fcn51 : TransferFcn  Commented=on  Denominator=[12 1]
  Transfer Fcn52 : TransferFcn  Commented=on  Denominator=[0.12 1]
  Transfer Fcn53 : TransferFcn  Commented=on  Denominator=[0.45 1]
  Transfer Fcn54 : TransferFcn  Commented=on  Denominator=[0.15 1]
  Transfer Fcn55 : TransferFcn  Commented=on  Denominator=[0.35 1]
  Transfer Fcn56 : TransferFcn  Commented=on  Denominator=[2*0.083 0.015]
  Transfer Fcn57 : TransferFcn  Commented=on  Denominator=[2*0.1 0.017]
  Transfer Fcn58 : TransferFcn  Commented=on  Denominator=[2*0.0623 0.014]
  Transfer Fcn59 : TransferFcn  Commented=on  Denominator=[2.73]
  Transfer Fcn6 : TransferFcn  Denominator=[2*0.083 0.015]
  Transfer Fcn7 : TransferFcn  Denominator=[2*0.1 0.017]
  Transfer Fcn8 : TransferFcn  Denominator=[2*0.0623 0.014]
  Transfer Fcn9 : TransferFcn  Denominator=[2.73]
  Uniform Random Number : UniformRandomNumber  Minimum=0.15  Maximum=0.25  SampleTime=25
  Uniform Random Number1 : UniformRandomNumber  Minimum=0.35  Maximum=0.40  SampleTime=25
  Uniform Random Number10 : UniformRandomNumber  Minimum=0.05  Maximum=0.075  SampleTime=10
  Uniform Random Number11 : UniformRandomNumber  Minimum=0.05  Maximum=0.075  SampleTime=10
  Uniform Random Number12 : UniformRandomNumber  Minimum=-0.01  Maximum=0.01  SampleTime=1
  Uniform Random Number13 : UniformRandomNumber  Minimum=-0.05  Maximum=0.05  SampleTime=1
  Uniform Random Number14 : UniformRandomNumber  Minimum=-0.01  Maximum=0.01  SampleTime=1
  Uniform Random Number15 : UniformRandomNumber  Minimum=-0.01  Maximum=0.01  SampleTime=1
  Uniform Random Number16 : UniformRandomNumber  Minimum=-0.015  Maximum=0.015  SampleTime=2
  Uniform Random Number17 : UniformRandomNumber  Minimum=-0.015  Maximum=0.015  SampleTime=2
  Uniform Random Number18 : UniformRandomNumber  Commented=on  Minimum=0.15  Maximum=0.25  SampleTime=25
  Uniform Random Number19 : UniformRandomNumber  Commented=on  Minimum=0.35  Maximum=0.40  SampleTime=25
  Uniform Random Number2 : UniformRandomNumber  Minimum=0.2  Maximum=0.30  SampleTime=3
  Uniform Random Number{20..21,38..39,56..57} (6 alike) : UniformRandomNumber  Commented=on  Minimum=0.05  Maximum=0.075  SampleTime=10
  Uniform Random Number{22,24..25,40,42..43,58,60..61} (9 alike) : UniformRandomNumber  Commented=on  Minimum=-0.01  Maximum=0.01  SampleTime=1
  Uniform Random Number23 : UniformRandomNumber  Commented=on  Minimum=-0.05  Maximum=0.05  SampleTime=1
  Uniform Random Number{26..27,44..45,62..63} (6 alike) : UniformRandomNumber  Commented=on  Minimum=-0.015  Maximum=0.015  SampleTime=2
  Uniform Random Number28 : UniformRandomNumber  Commented=on  Minimum=0.2  Maximum=0.30  SampleTime=3
  Uniform Random Number29 : UniformRandomNumber  Commented=on  Minimum=0.225  Maximum=0.275  SampleTime=5
  Uniform Random Number3 : UniformRandomNumber  Minimum=0.225  Maximum=0.275  SampleTime=5
  Uniform Random Number30 : UniformRandomNumber  Commented=on  Minimum=0.15  Maximum=0.2  SampleTime=15
  Uniform Random Number31 : UniformRandomNumber  Commented=on  Minimum=0.075  Maximum=0.10  SampleTime=15
  Uniform Random Number{32..33,50..51,68..69} (6 alike) : UniformRandomNumber  Commented=on  Minimum=0.10  Maximum=0.15  SampleTime=20
  Uniform Random Number34 : UniformRandomNumber  Commented=on  Minimum=0.125  Maximum=0.15  SampleTime=15
  Uniform Random Number35 : UniformRandomNumber  Commented=on  Minimum=0.05  Maximum=0.10  SampleTime=15
  Uniform Random Number36 : UniformRandomNumber  Commented=on  Minimum=0.15  Maximum=0.25  SampleTime=25
  Uniform Random Number37 : UniformRandomNumber  Commented=on  Minimum=0.35  Maximum=0.40  SampleTime=25
  Uniform Random Number4 : UniformRandomNumber  Minimum=0.15  Maximum=0.2  SampleTime=15
  Uniform Random Number41 : UniformRandomNumber  Commented=on  Minimum=-0.05  Maximum=0.05  SampleTime=1
  Uniform Random Number46 : UniformRandomNumber  Commented=on  Minimum=0.2  Maximum=0.30  SampleTime=3
  Uniform Random Number47 : UniformRandomNumber  Commented=on  Minimum=0.225  Maximum=0.275  SampleTime=5
  Uniform Random Number48 : UniformRandomNumber  Commented=on  Minimum=0.15  Maximum=0.2  SampleTime=15
  Uniform Random Number49 : UniformRandomNumber  Commented=on  Minimum=0.075  Maximum=0.10  SampleTime=15
  Uniform Random Number5 : UniformRandomNumber  Minimum=0.075  Maximum=0.10  SampleTime=15
  Uniform Random Number52 : UniformRandomNumber  Commented=on  Minimum=0.125  Maximum=0.15  SampleTime=15
  Uniform Random Number53 : UniformRandomNumber  Commented=on  Minimum=0.05  Maximum=0.10  SampleTime=15
  Uniform Random Number54 : UniformRandomNumber  Commented=on  Minimum=0.15  Maximum=0.25  SampleTime=25
  Uniform Random Number55 : UniformRandomNumber  Commented=on  Minimum=0.35  Maximum=0.40  SampleTime=25
  Uniform Random Number59 : UniformRandomNumber  Commented=on  Minimum=-0.05  Maximum=0.05  SampleTime=1
  Uniform Random Number6 : UniformRandomNumber  Minimum=0.10  Maximum=0.15  SampleTime=20
  Uniform Random Number64 : UniformRandomNumber  Commented=on  Minimum=0.2  Maximum=0.30  SampleTime=3
  Uniform Random Number65 : UniformRandomNumber  Commented=on  Minimum=0.225  Maximum=0.275  SampleTime=5
  Uniform Random Number66 : UniformRandomNumber  Commented=on  Minimum=0.15  Maximum=0.2  SampleTime=15
  Uniform Random Number67 : UniformRandomNumber  Commented=on  Minimum=0.075  Maximum=0.10  SampleTime=15
  Uniform Random Number7 : UniformRandomNumber  Minimum=0.10  Maximum=0.15  SampleTime=20
  Uniform Random Number70 : UniformRandomNumber  Commented=on  Minimum=0.125  Maximum=0.15  SampleTime=15
  Uniform Random Number71 : UniformRandomNumber  Commented=on  Minimum=0.05  Maximum=0.10  SampleTime=15
  Uniform Random Number8 : UniformRandomNumber  Minimum=0.125  Maximum=0.15  SampleTime=15
  Uniform Random Number9 : UniformRandomNumber  Minimum=0.05  Maximum=0.10  SampleTime=15
  VIC : Scope  NumInputPorts=3
  VIC1 : Scope  NumInputPorts=3
  Wind1 : TransferFcn  Denominator=[1.85 1]
  Wind10 : TransferFcn  Commented=on  Denominator=[1.85 1]
  Wind11 : TransferFcn  Commented=on  Denominator=[1.55 1]
  Wind12 : TransferFcn  Commented=on  Denominator=[1.95 1]
  Wind2 : TransferFcn  Denominator=[1.55 1]
  Wind3 : TransferFcn  Denominator=[1.95 1]
  Wind4 : TransferFcn  Commented=on  Denominator=[1.85 1]
  Wind5 : TransferFcn  Commented=on  Denominator=[1.55 1]
  Wind6 : TransferFcn  Commented=on  Denominator=[1.95 1]
  Wind7 : TransferFcn  Commented=on  Denominator=[1.85 1]
  Wind8 : TransferFcn  Commented=on  Denominator=[1.55 1]
  Wind9 : TransferFcn  Commented=on  Denominator=[1.95 1]
  wires:
  Sum1/1 -> Transfer Fcn7/1
  Sum2/1 -> Transfer Fcn8/1
  Sum/1 -> Transfer Fcn6/1
  Integrator/1 -> Gain8/1
  Sum5/1 -> Transfer Fcn/1
  Sum3/1 -> Transfer Fcn2/1
  Integrator1/1 -> Gain3/1
  Integrator2/1 -> Gain2/1
  Sum4/1 -> Transfer Fcn4/1
  Transfer Fcn9/1 -> Sum3/1
  Transfer Fcn10/1 -> Sum5/1
  Transfer Fcn11/1 -> Sum4/1
  Gain5/1 -> Sum11/1
  Gain/1 -> Sum11/2
  Gain4/1 -> Sum10/2
  Gain1/1 -> Sum10/1
  Gain3/1 -> Sum3/2
  Gain2/1 -> Sum4/2
  Gain6/1 -> Sum9/1
  Gain7/1 -> Sum9/2
  Gain8/1 -> Sum5/2
  Transfer Fcn14/1 -> Saturation1/1
  Saturation2/1 -> VIC/2, Sum1/3, Scope4/1
  Transfer Fcn12/1 -> Saturation/1
  Sum15/1 -> PowerPlant1/1, Sum1/1, To Workspace4/1
  Sum16/1 -> Sum/1, PowerPlant2/1, To Workspace3/1
  Sum17/1 -> To Workspace5/1, Sum2/1, PowerPlant3/1
  Uniform Random Number/1 -> First Order Hold5/1
  Uniform Random Number1/1 -> First Order Hold7/1
  Uniform Random Number2/1 -> First Order Hold4/1
  Uniform Random Number3/1 -> First Order Hold1/1
  Uniform Random Number4/1 -> First Order Hold3/1
  Uniform Random Number5/1 -> First Order Hold2/1
  Uniform Random Number6/1 -> First Order Hold15/1
  Uniform Random Number7/1 -> First Order Hold16/1
  Transfer Fcn1/1 -> Sum18/1, PowerPlant2/2
  Transfer Fcn3/1 -> PowerPlant1/2, Sum20/1
  Sum21/1 -> Sum20/2, PowerPlant1/3, To Workspace6/1
  Uniform Random Number8/1 -> First Order Hold14/1
  Uniform Random Number9/1 -> First Order Hold13/1
  Transfer Fcn5/1 -> PowerPlant3/2, Sum23/1
  Transfer Fcn13/1 -> Saturation2/1
  Saturation1/1 -> Sum2/3, Scope5/1, VIC/3
  Saturation/1 -> Sum/3, Scope3/1, VIC/1
  Wind3/1 -> Sum22/2
  Solar3/1 -> Sum22/1
  Solar2/1 -> Sum21/1
  Wind2/1 -> Sum21/2
  Wind1/1 -> Sum19/2
  Solar1/1 -> Sum19/1
  GRC/1 -> Limiter2/1
  Transfer Fcn/1 -> GRC/1
  Limiter2/1 -> Transfer Fcn1/1
  Deadband/1 -> GRC11/1
  Transfer Fcn2/1 -> Deadband/1
  GRC11/1 -> Transfer Fcn3/1
  GRC2/1 -> Limiter3/1
  Limiter3/1 -> Transfer Fcn5/1
  Transfer Fcn4/1 -> GRC2/1
  Sum18/1 -> Sum12/1
  Sum12/1 -> Sum/2
  Sum20/1 -> Sum13/1
  Sum13/1 -> Sum1/2
  Sum23/1 -> Sum14/1
  Sum14/1 -> Sum2/2
  Transfer Fcn6/1 -> Gain12/1, Derivative3/1, Agent 1/1(error), Sum24/1, Transfer Fcn10/1, Gain1/1, Gain5/1, Abs/1, VIC1/1, To Workspace/1
  Sum8/1 -> Gain9/1
  Sum7/1 -> Gain10/1
  Sum6/1 -> Gain11/1
  First Order Hold7/1 -> Sum27/1
  Sum27/1 -> Sum16/2
  First Order Hold8/1 -> Sum27/2
  Industrial Loads1/1 -> First Order Hold8/1
  Sum28/1 -> Sum16/1
  First Order Hold5/1 -> Sum28/1
  First Order Hold6/1 -> Sum28/2
  Industrial Loads2/1 -> First Order Hold6/1
  First Order Hold9/1 -> Sum29/2
  Uniform Random Number12/1 -> First Order Hold9/1
  Uniform Random Number11/1 -> First Order Hold12/1
  Sum29/1 -> Wind3/1
  Uniform Random Number10/1 -> First Order Hold11/1
  Sum30/1 -> Solar3/1
  First Order Hold10/1 -> Sum30/2
  Uniform Random Number13/1 -> First Order Hold10/1
  First Order Hold11/1 -> Sum30/1
  First Order Hold12/1 -> Sum29/1
  First Order Hold17/1 -> Sum31/2
  Industrial Loads3/1 -> First Order Hold17/1
  First Order Hold1/1 -> Sum31/1
  Industrial Loads4/1 -> First Order Hold18/1
  First Order Hold18/1 -> Sum32/2
  First Order Hold4/1 -> Sum32/1
  Sum32/1 -> Sum15/1
  First Order Hold19/1 -> Sum33/2
  Industrial Loads5/1 -> First Order Hold19/1
  First Order Hold2/1 -> Sum33/1
  Sum33/1 -> Sum17/2
  First Order Hold20/1 -> Sum34/2
  Industrial Loads6/1 -> First Order Hold20/1
  Sum34/1 -> Sum17/1
  First Order Hold3/1 -> Sum34/1
  Manual Variant Source7/1 -> Sum12/2, Sum24/2
  Manual Variant Source11/1 -> Sum26/2, Sum14/2
  Manual Variant Source9/1 -> Sum25/2, Sum13/2
  Gain9/1 -> Integrator4/1
  Gain10/1 -> Integrator5/1
  Gain11/1 -> Integrator3/1
  Gain12/1 -> Sum8/1
  Gain13/1 -> Sum7/1
  Gain14/1 -> Sum6/1
  Sum35/1 -> Solar1/1
  First Order Hold15/1 -> Sum35/1
  Sum36/1 -> Wind1/1
  First Order Hold16/1 -> Sum36/1
  Sum37/1 -> Solar2/1
  Sum38/1 -> Wind2/1
  First Order Hold14/1 -> Sum37/1
  First Order Hold13/1 -> Sum38/1
  Uniform Random Number14/1 -> First Order Hold21/1
  First Order Hold21/1 -> Sum38/2
  Uniform Random Number15/1 -> First Order Hold22/1
  First Order Hold22/1 -> Sum37/2
  First Order Hold23/1 -> Sum36/2
  Uniform Random Number16/1 -> First Order Hold23/1
  Uniform Random Number17/1 -> First Order Hold24/1
  First Order Hold24/1 -> Sum35/2
  Integrator8/1 -> To Workspace11/1, Display/1
  Integrator6/1 -> To Workspace10/1, Display1/1
  Abs2/1 -> Integrator7/1
  Manual Variant Source4/1 -> Transfer Fcn13/1
  Manual Variant Source5/1 -> Transfer Fcn14/1
  Manual Variant Source3/1 -> Transfer Fcn12/1
  Gain16/1 -> Manual Variant Source4/2
  Gain17/1 -> Manual Variant Source3/2
  Derivative3/1 -> Gain17/1, Product/2
  Derivative1/1 -> Gain16/1, Product1/2
  Derivative2/1 -> Gain15/1, Product2/2
  Transfer Fcn7/1 -> Gain6/1, Agent 2/1(error), Derivative1/1, Transfer Fcn9/1, Sum25/1, Gain13/1, Gain/1, Abs1/1, VIC1/2, To Workspace1/1
  Product/1 -> Manual Variant Source3/1
  Product2/1 -> Manual Variant Source5/1, Scope2/1
  Gain15/1 -> Manual Variant Source5/2
  Sum9/1 -> Sum8/2
  Sum10/1 -> Sum7/2
  Sum11/1 -> Sum6/2
  Sum31/1 -> Sum15/2
  Abs/1 -> Integrator8/1
  Integrator7/1 -> Display2/1, To Workspace9/1
  Abs1/1 -> Integrator6/1
  Integrator5/1 -> Manual Variant Source6/2, Product3/2
  Integrator3/1 -> Manual Variant Source8/1, Product4/1
  Integrator4/1 -> Manual Variant Source10/1, Product5/1
  Transfer Fcn8/1 -> Sum26/1, Transfer Fcn11/1, VIC1/3, To Workspace2/1, Abs2/1, Gain7/1, Gain4/1, Agent 3/1(error), Derivative2/1, Gain14/1
  Sum22/1 -> PowerPlant3/3, To Workspace8/1, Sum23/2
  Product3/1 -> Manual Variant Source6/1
  Product5/1 -> Manual Variant Source10/2
  Step/1 -> Product5/2
  Step1/1 -> Product3/1
  Step2/1 -> Product4/2
  Agent 1/1(Action) -> Scope/1, Product/1
  Agent 2/1(Action) -> Product1/1
  Agent 3/1(Action) -> Product2/1
  Product1/1 -> Scope1/1, Manual Variant Source4/1
  Product4/1 -> Manual Variant Source8/2
  Sum24/1 -> Integrator/1
  Sum25/1 -> Integrator1/1
  Sum26/1 -> Integrator2/1
  Integrator9/1 -> Reward1/1
  Constant2/1 -> Integrator9/1
  Manual Variant Source10/1 -> Manual Variant Source7/1
  Manual Variant Source6/1 -> Manual Variant Source9/1
  Manual Variant Source8/1 -> Manual Variant Source11/1
  Manual Variant Source14/1 -> Manual Variant Source21/1
  Integrator15/1 -> Manual Variant Source20/2, Product9/2
  Sum57/1 -> Integrator11/1
  First Order Hold27/1 -> Sum63/1
  Manual Variant Source22/1 -> Manual Variant Source15/1
  First Order Hold47/1 -> Sum59/2
  Uniform Random Number22/1 -> First Order Hold48/1
  Uniform Random Number18/1 -> First Order Hold44/1
  Sum65/1 -> Sum46/1
  Product10/1 -> Manual Variant Source22/2
  Transfer Fcn29/1 -> Sum62/1
  GRC4/1 -> Limiter4/1
  Sum56/1 -> Integrator10/1
  Manual Variant Source23/1 -> Sum57/2, Sum44/2
  Gain28/1 -> Sum72/2
  Sum55/1 -> Sum45/1
  Step5/1 -> Product10/2
  Integrator14/1 -> Manual Variant Source14/1, Product11/1
  First Order Hold32/1 -> Sum69/1
  Uniform Random Number25/1 -> First Order Hold39/1
  Sum52/1 -> Sum44/1
  First Order Hold46/1 -> Sum59/1
  First Order Hold40/1 -> Sum69/2
  Derivative6/1 -> Product6/2
  Product7/1 -> Transfer Fcn20/1, Scope7/1
  Sum76/1 -> Gain35/1
  Step3/1 -> Product11/2
  Uniform Random Number32/1 -> First Order Hold31/1
  Gain18/1 -> Sum42/2
  Uniform Random Number33/1 -> First Order Hold32/1
  First Order Hold45/1 -> Sum60/2
  Transfer Fcn22/1 -> GRC4/1
  First Order Hold25/1 -> Sum64/1
  Uniform Random Number24/1 -> First Order Hold38/1
  First Order Hold39/1 -> Sum70/2
  Gain19/1 -> Sum41/1
  Product9/1 -> Manual Variant Source20/1
  Derivative5/1 -> Product8/2
  First Order Hold41/1 -> Sum68/2
  Sum54/1 -> Sum55/2
  Product11/1 -> Manual Variant Source14/2
  Sum77/1 -> Sum76/2
  Uniform Random Number34/1 -> First Order Hold30/1
  Product6/1 -> Transfer Fcn19/1, Scope6/1
  First Order Hold38/1 -> Sum71/2
  Sum40/1 -> Transfer Fcn27/1
  Saturation3/1 -> Sum39/3, Scope9/1
  Sum63/1 -> Solar6/1
  Solar4/1 -> Sum50/1
  Product8/1 -> Transfer Fcn21/1, Scope8/1
  Integrator13/1 -> Manual Variant Source22/1, Product10/1
  Gain23/1 -> Sum75/1
  Integrator10/1 -> Gain34/1
  Gain21/1 -> Integrator13/1
  Sum67/1 -> Sum48/1
  First Order Hold30/1 -> Sum70/1
  First Order Hold48/1 -> Sum61/2
  First Order Hold29/1 -> Sum71/1
  Gain31/1 -> Sum42/1
  Sum68/1 -> Solar4/1
  Industrial Loads7/1 -> First Order Hold47/1
  First Order Hold31/1 -> Sum68/1
  Gain24/1 -> Sum74/1
  First Order Hold34/1 -> Sum65/2
  First Order Hold43/1 -> Sum65/1
  Sum69/1 -> Wind4/1
  Industrial Loads12/1 -> First Order Hold37/1
  First Order Hold37/1 -> Sum67/2
  Transfer Fcn19/1 -> Saturation3/1
  Gain20/1 -> Integrator15/1
  Transfer Fcn18/1 -> Sum72/1
  Transfer Fcn16/1 -> Sum49/1, PowerPlant4/2
  First Order Hold35/1 -> Sum66/2
  Gain22/1 -> Sum76/1
  Gain35/1 -> Integrator14/1
  Sum42/1 -> Sum74/2
  Manual Variant Source15/1 -> Sum58/2, Sum45/2
  Industrial Loads11/1 -> First Order Hold35/1
  First Order Hold36/1 -> Sum66/1
  Industrial Loads10/1 -> First Order Hold34/1
  First Order Hold33/1 -> Sum64/2
  First Order Hold26/1 -> Sum63/2
  Derivative4/1 -> Product7/2
  Uniform Random Number23/1 -> First Order Hold26/1
  First Order Hold28/1 -> Sum61/1
  Integrator11/1 -> Gain29/1
  Sum61/1 -> Wind6/1
  Industrial Loads8/1 -> First Order Hold45/1
  First Order Hold44/1 -> Sum60/1
  Sum48/1 -> Sum51/1
  Sum75/1 -> Gain20/1
  Sum64/1 -> Sum46/2
  Sum44/1 -> Sum40/2
  Limiter6/1 -> Transfer Fcn25/1
  Sum66/1 -> Sum48/2
  Solar5/1 -> Sum53/1
  Uniform Random Number19/1 -> First Order Hold46/1
  Uniform Random Number26/1 -> First Order Hold40/1
  Limiter5/1 -> Transfer Fcn16/1
  Limiter4/1 -> Transfer Fcn23/1
  Wind4/1 -> Sum50/2
  Wind6/1 -> Sum54/2
  Transfer Fcn20/1 -> Saturation5/1
  Transfer Fcn15/1 -> GRC3/1
  Uniform Random Number20/1 -> First Order Hold27/1
  Wind5/1 -> Sum53/2
  Transfer Fcn25/1 -> Sum55/1
  Manual Variant Source21/1 -> Sum56/2, Sum43/2
  Sum41/1 -> Sum75/2
  Sum62/1 -> Transfer Fcn22/1
  Solar6/1 -> Sum54/1
  GRC3/1 -> Limiter5/1
  Sum47/1 -> Sum39/1, PowerPlant4/1, To Workspace12/1
  Sum74/1 -> Gain21/1
  Sum71/1 -> Wind5/1
  Transfer Fcn21/1 -> Saturation4/1
  Saturation5/1 -> Sum40/3, Scope10/1
  Step4/1 -> Product9/1
  Gain34/1 -> Sum73/2
  Uniform Random Number35/1 -> First Order Hold29/1
  Sum43/1 -> Sum39/2
  Sum58/1 -> Integrator12/1
  Uniform Random Number31/1 -> First Order Hold36/1
  Uniform Random Number29/1 -> First Order Hold25/1
  Sum53/1 -> Sum52/2
  Gain33/1 -> Sum77/2
  Transfer Fcn23/1 -> Sum52/1
  Sum59/1 -> Sum47/2
  Transfer Fcn24/1 -> GRC5/1
  Transfer Fcn17/1 -> Sum73/1
  Uniform Random Number21/1 -> First Order Hold28/1
  Sum46/1 -> Sum40/1
  Uniform Random Number28/1 -> First Order Hold43/1
  Saturation4/1 -> Sum51/3, Scope11/1
  Gain29/1 -> Sum62/2
  Sum73/1 -> Transfer Fcn15/1
  Integrator12/1 -> Gain28/1
  Sum39/1 -> Transfer Fcn26/1
  Sum49/1 -> Sum43/1
  Gain30/1 -> Sum41/2
  Sum45/1 -> Sum51/2
  Industrial Loads9/1 -> First Order Hold33/1
  Sum51/1 -> Transfer Fcn28/1
  GRC5/1 -> Limiter6/1
  Sum60/1 -> Sum47/1
  Uniform Random Number27/1 -> First Order Hold41/1
  Gain32/1 -> Sum77/1
  Sum70/1 -> Solar5/1
  Uniform Random Number30/1 -> First Order Hold42/1
  First Order Hold42/1 -> Sum67/1
  Sum72/1 -> Transfer Fcn24/1
  Manual Variant Source20/1 -> Manual Variant Source23/1
  Integrator18/1 -> Display3/1
  Abs5/1 -> Integrator17/1
  Abs3/1 -> Integrator18/1
  Abs4/1 -> Integrator16/1
  Integrator16/1 -> Display4/1
  Integrator17/1 -> Display5/1
  Sum19/1 -> Sum18/2, PowerPlant2/3, To Workspace7/1
  First Order Hold70/1 -> Sum98/1
  Transfer Fcn35/1 -> Saturation8/1
  First Order Hold67/1 -> Sum104/1
  Integrator25/1 -> Display7/1
  Integrator26/1 -> Display8/1
  Integrator22/1 -> Manual Variant Source17/1, Product12/1
  Transfer Fcn34/1 -> Saturation6/1
  Uniform Random Number46/1 -> First Order Hold67/1
  Saturation7/1 -> Sum90/3, Scope13/1
  Uniform Random Number48/1 -> First Order Hold66/1
  Abs6/1 -> Integrator27/1
  Abs7/1 -> Integrator25/1
  Solar7/1 -> Sum89/1
  Integrator27/1 -> Display6/1
  Sum111/1 -> Transfer Fcn39/1
  Uniform Random Number53/1 -> First Order Hold53/1
  First Order Hold66/1 -> Sum106/1
  Sum90/1 -> Transfer Fcn43/1
  Sum78/1 -> Transfer Fcn41/1
  First Order Hold55/1 -> Sum107/1
  Gain44/1 -> Sum116/1
  Sum109/1 -> Solar8/1
  Gain45/1 -> Sum116/2
  Product12/1 -> Manual Variant Source17/2
  Sum87/1 -> Sum90/1
  Transfer Fcn39/1 -> GRC7/1
  Sum84/1 -> Sum90/2
  First Order Hold72/1 -> Sum100/2
  GRC7/1 -> Limiter8/1
  Industrial Loads18/1 -> First Order Hold57/1
  Gain42/1 -> Sum80/2
  First Order Hold61/1 -> Sum106/2
  Integrator21/1 -> Gain40/1
  Sum92/1 -> Sum91/2
  Sum88/1 -> Sum82/1
  PID Controller3/1 -> Product16/1
  Sum114/1 -> Gain27/1
  Step8/1 -> Product12/2
  Sum112/1 -> Transfer Fcn30/1
  First Order Hold62/1 -> Sum110/2
  Industrial Loads13/1 -> First Order Hold58/1
  Sum85/1 -> Sum79/1
  Integrator20/1 -> Gain41/1
  Uniform Random Number39/1 -> First Order Hold52/1
  Sum81/1 -> Sum113/2
  Uniform Random Number49/1 -> First Order Hold60/1
  First Order Hold60/1 -> Sum105/1
  Uniform Random Number47/1 -> First Order Hold49/1
  Sum98/1 -> Sum86/2
  Saturation8/1 -> Sum79/3, Scope12/1
  Manual Variant Source16/1 -> Sum95/2, Sum82/2
  Transfer Fcn32/1 -> Sum112/1
  Sum113/1 -> Gain36/1
  Sum82/1 -> Sum78/2
  Solar8/1 -> Sum92/1
  Step7/1 -> Product17/1
  Integrator19/1 -> Gain46/1
  Sum101/1 -> Transfer Fcn37/1
  Industrial Loads14/1 -> First Order Hold59/1
  Wind7/1 -> Sum89/2
  First Order Hold51/1 -> Sum102/1
  Wind9/1 -> Sum93/2
  Limiter1/1 -> Transfer Fcn38/1
  Sum110/1 -> Wind8/1
  Sum105/1 -> Sum87/2
  Gain25/1 -> Sum81/2
  Sum80/1 -> Sum114/2
  Sum96/1 -> Integrator20/1
  Transfer Fcn40/1 -> Sum94/1
  First Order Hold64/1 -> Sum108/2
  Sum86/1 -> Sum78/1, PowerPlant5/1, To Workspace13/1
  Uniform Random Number45/1 -> First Order Hold65/1
  Solar9/1 -> Sum93/1
  GRC1/1 -> Limiter7/1
  Wind8/1 -> Sum92/2
  Limiter7/1 -> Transfer Fcn31/1
  Industrial Loads17/1 -> First Order Hold69/1
  Limiter8/1 -> Transfer Fcn40/1
  Uniform Random Number44/1 -> First Order Hold64/1
  Transfer Fcn31/1 -> Sum88/1, PowerPlant5/2
  Sum83/1 -> Sum79/2
  Derivative7/1 -> Product15/2
  First Order Hold50/1 -> Sum102/2
  Manual Variant Source18/1 -> Sum96/2, Sum83/2
  Uniform Random Number41/1 -> First Order Hold50/1
  Transfer Fcn30/1 -> GRC1/1
  First Order Hold57/1 -> Sum103/2
  GRC6/1 -> Limiter1/1
  Manual Variant Source12/1 -> Sum97/2, Sum84/2
  Gain46/1 -> Sum112/2
  Sum108/1 -> Wind7/1
  First Order Hold63/1 -> Sum109/2
  Gain37/1 -> Sum115/1
  Gain47/1 -> Integrator23/1
  First Order Hold59/1 -> Sum105/2
  Sum106/1 -> Sum87/1
  Transfer Fcn33/1 -> Sum111/1
  Gain27/1 -> Integrator24/1
  Industrial Loads15/1 -> First Order Hold61/1
  Product13/1 -> Manual Variant Source2/2
  Gain43/1 -> Sum81/1
  Industrial Loads16/1 -> First Order Hold71/1
  Gain36/1 -> Integrator22/1
  First Order Hold58/1 -> Sum104/2
  Product16/1 -> Transfer Fcn36/1, Scope16/1
  Gain39/1 -> Sum113/1
  First Order Hold53/1 -> Sum110/1
  Gain38/1 -> Sum114/1
  Sum102/1 -> Solar9/1
  First Order Hold68/1 -> Sum99/1
  Sum116/1 -> Sum115/2
  Sum93/1 -> Sum94/2
  Sum95/1 -> Integrator19/1
  Saturation6/1 -> Sum78/3, Scope17/1
  Sum104/1 -> Sum85/1
  Product14/1 -> Transfer Fcn34/1, Scope14/1
  Uniform Random Number52/1 -> First Order Hold54/1
  Sum97/1 -> Integrator21/1
  First Order Hold65/1 -> Sum107/2
  Sum107/1 -> Solar7/1
  Transfer Fcn37/1 -> GRC6/1
  First Order Hold71/1 -> Sum98/2
  Derivative8/1 -> Product16/2
  PID Controller1/1 -> Product15/1
  First Order Hold49/1 -> Sum103/1
  Product17/1 -> Manual Variant Source13/1
  Gain26/1 -> Sum80/1
  Uniform Random Number42/1 -> First Order Hold62/1
  Uniform Random Number50/1 -> First Order Hold55/1
  First Order Hold69/1 -> Sum99/2
  Integrator23/1 -> Manual Variant Source2/1, Product13/1
  Uniform Random Number51/1 -> First Order Hold56/1
  First Order Hold52/1 -> Sum100/1
  First Order Hold54/1 -> Sum109/1
  Product15/1 -> Transfer Fcn35/1, Scope15/1
  Gain40/1 -> Sum111/2
  First Order Hold56/1 -> Sum108/1
  Sum91/1 -> Sum83/1
  Sum94/1 -> Sum84/1
  Uniform Random Number36/1 -> First Order Hold68/1
  Uniform Random Number40/1 -> First Order Hold72/1
  Step6/1 -> Product13/2
  Manual Variant Source2/1 -> Manual Variant Source16/1
  Manual Variant Source17/1 -> Manual Variant Source12/1
  Sum79/1 -> Transfer Fcn42/1
  PID Controller2/1 -> Product14/1
  Transfer Fcn38/1 -> Sum91/1
  Sum99/1 -> Sum86/1
  Gain41/1 -> Sum101/2
  Uniform Random Number37/1 -> First Order Hold70/1
  Transfer Fcn36/1 -> Saturation7/1
  Sum100/1 -> Wind9/1
  Abs8/1 -> Integrator26/1
  Derivative9/1 -> Product14/2
  Sum115/1 -> Gain47/1
  Transfer Fcn41/1 -> Gain37/1, Derivative9/1, PID Controller2/1, Frequency/2, Abs6/1, Sum95/1, Transfer Fcn32/1, Gain26/1, Gain43/1
  Manual Variant Source13/1 -> Manual Variant Source18/1
  Uniform Random Number38/1 -> First Order Hold51/1
  Sum89/1 -> Sum88/2, PowerPlant5/3
  Transfer Fcn44/1 -> Sum101/1
  Sum103/1 -> Sum85/2
  Integrator24/1 -> Manual Variant Source13/2, Product17/2
  Uniform Random Number43/1 -> First Order Hold63/1
  Mux1/1 -> Fuzzy Logic Controller1/1
  Fuzzy Logic Controller1/1 -> Product6/1
  Fuzzy Logic Controller2/1 -> Product7/1
  Mux2/1 -> Fuzzy Logic Controller2/1
  Fuzzy Logic Controller3/1 -> Product8/1
  Mux3/1 -> Fuzzy Logic Controller3/1
  Sum50/1 -> PowerPlant4/3, Sum49/2
  Gain58/1 -> Sum118/2
  Transfer Fcn53/1 -> Sum147/1
  Sum135/1 -> Transfer Fcn57/1
  Step9/1 -> Product19/2
  Manual Variant Source28/1 -> Manual Variant Source25/1
  Uniform Random Number54/1 -> First Order Hold92/1
  Uniform Random Number58/1 -> First Order Hold96/1
  Product21/1 -> Transfer Fcn50/1, Scope21/1
  First Order Hold80/1 -> Sum125/1
  Sum150/1 -> Sum140/1
  First Order Hold76/1 -> Sum117/1
  First Order Hold73/1 -> Sum120/1
  First Order Hold93/1 -> Sum155/2
  Uniform Random Number69/1 -> First Order Hold80/1
  Transfer Fcn58/1 -> PowerPlant7/3, Abs11/1, Sum153/1, Transfer Fcn48/1, Gain62/1, Gain59/1, MPC Controller2/1, Derivative11/1, Gain56/1
  Uniform Random Number55/1 -> First Order Hold94/1
  Derivative11/1 -> Product22/2
  MPC Controller/1 -> Product20/1
  First Order Hold95/1 -> Sum154/2
  Sum151/1 -> Integrator28/1
  Sum153/1 -> Integrator30/1
  Integrator32/1 -> Manual Variant Source28/1, Product19/1
  Transfer Fcn52/1 -> GRC9/1
  Uniform Random Number70/1 -> First Order Hold78/1
  Product20/1 -> Scope20/1, Transfer Fcn49/1
  Product23/1 -> Manual Variant Source24/1
  Sum149/1 -> MPC Controller2/3, Sum150/2
  Sum124/1 -> Solar10/1
  First Order Hold89/1 -> Sum124/2
  Gain57/1 -> Sum128/2
  Industrial Loads22/1 -> First Order Hold95/1
  Product19/1 -> Manual Variant Source28/2
  First Order Hold82/1 -> Sum121/2
  Gain53/1 -> Integrator31/1
  Sum123/1 -> Sum143/1
  Transfer Fcn48/1 -> Sum128/1
  Manual Variant Source19/1 -> Sum153/2, Sum140/2
  Gain56/1 -> Sum130/1
  Industrial Loads21/1 -> First Order Hold85/1
  Gain63/1 -> Sum129/2
  Sum125/1 -> Wind10/1
  Gain51/1 -> Integrator33/1
  Gain64/1 -> Integrator32/1
  First Order Hold87/1 -> Sum126/2
  Uniform Random Number59/1 -> First Order Hold74/1
  First Order Hold81/1 -> Sum120/2
  First Order Hold77/1 -> Sum127/1
  Manual Variant Source27/1 -> Sum152/2, Sum139/2
  Uniform Random Number62/1 -> First Order Hold88/1
  Limiter11/1 -> Transfer Fcn55/1
  GRC9/1 -> Limiter9/1
  Transfer Fcn45/1 -> GRC8/1
  Sum152/1 -> Integrator29/1
  Sum142/1 -> Sum134/1, PowerPlant6/1, To Workspace14/1
  Transfer Fcn55/1 -> Sum150/1
  Transfer Fcn51/1 -> Saturation10/1
  Uniform Random Number63/1 -> First Order Hold89/1
  Solar12/1 -> Sum149/1
  Uniform Random Number60/1 -> First Order Hold86/1
  Wind11/1 -> Sum148/2
  First Order Hold88/1 -> Sum125/2
  Integrator28/1 -> Gain63/1
  Wind12/1 -> Sum149/2
  Sum122/1 -> Sum143/2
  MPC Controller1/1 -> Product21/1
  Sum127/1 -> Wind11/1
  Limiter9/1 -> Transfer Fcn53/1
  Solar11/1 -> Sum148/1
  First Order Hold75/1 -> Sum119/1
  Industrial Loads20/1 -> First Order Hold83/1
  Step10/1 -> Product23/1
  Gain55/1 -> Sum131/1
  Gain50/1 -> Sum136/1
  Sum118/1 -> Transfer Fcn52/1
  Wind10/1 -> Sum145/2
  Sum154/1 -> Sum142/2
  Uniform Random Number67/1 -> First Order Hold84/1
  First Order Hold83/1 -> Sum122/2
  First Order Hold74/1 -> Sum119/2
  Saturation11/1 -> Sum135/3, Scope18/1
  First Order Hold84/1 -> Sum122/1
  Transfer Fcn47/1 -> Sum129/1
  Transfer Fcn57/1 -> Derivative10/1, Gain61/1, MPC Controller1/1, Transfer Fcn59/1, Sum152/1, PowerPlant7/2, Abs10/1, Gain55/1, Gain49/1
  Industrial Loads23/1 -> First Order Hold93/1
  Gain60/1 -> Sum137/1
  Sum133/1 -> Sum132/2
  Uniform Random Number65/1 -> First Order Hold73/1
  Sum141/1 -> Sum135/1
  Saturation9/1 -> Sum134/3, Scope23/1
  Integrator29/1 -> Gain58/1
  Limiter10/1 -> Transfer Fcn46/1
  Sum139/1 -> Sum135/2
  Product22/1 -> Transfer Fcn51/1, Scope22/1
  Sum137/1 -> Sum130/2
  Uniform Random Number57/1 -> First Order Hold76/1
  Integrator30/1 -> Gain57/1
  First Order Hold85/1 -> Sum123/2
  Sum131/1 -> Gain51/1
  Sum144/1 -> Sum138/1
  Sum130/1 -> Gain53/1
  Sum129/1 -> Transfer Fcn45/1
  Industrial Loads24/1 -> First Order Hold81/1
  MPC Controller2/1 -> Product22/1
  Gain59/1 -> Sum136/2
  GRC10/1 -> Limiter11/1
  GRC8/1 -> Limiter10/1
  Sum148/1 -> MPC Controller1/3, Sum147/2
  Industrial Loads19/1 -> First Order Hold82/1
  Step11/1 -> Product18/2
  First Order Hold86/1 -> Sum127/2
  Derivative10/1 -> Product21/2
  Gain62/1 -> Sum133/2
  Product18/1 -> Manual Variant Source26/2
  Sum143/1 -> Sum146/1
  First Order Hold90/1 -> Sum123/1
  Sum126/1 -> Solar11/1
  First Order Hold79/1 -> Sum124/1
  Sum134/1 -> Transfer Fcn56/1
  Gain61/1 -> Sum133/1
  Manual Variant Source25/1 -> Sum151/2, Sum138/2
  Sum146/1 -> Transfer Fcn58/1
  Sum121/1 -> Sum141/1
  Solar10/1 -> Sum145/1
  Sum140/1 -> Sum146/2
  Abs10/1 -> Integrator34/1
  Abs9/1 -> Integrator36/1
  Uniform Random Number66/1 -> First Order Hold90/1
  Transfer Fcn49/1 -> Saturation9/1
  Gain54/1 -> Sum132/1
  Saturation10/1 -> Sum146/3, Scope19/1
  Sum155/1 -> Sum142/1
  Integrator36/1 -> Display9/1
  Sum128/1 -> Transfer Fcn54/1
  Sum136/1 -> Sum131/2
  First Order Hold91/1 -> Sum121/1
  Transfer Fcn50/1 -> Saturation11/1
  Uniform Random Number71/1 -> First Order Hold77/1
  Transfer Fcn46/1 -> Sum144/1, PowerPlant6/2
  Abs11/1 -> Integrator35/1
  Gain49/1 -> Sum137/2
  Uniform Random Number68/1 -> First Order Hold79/1
  First Order Hold96/1 -> Sum117/2
  Sum132/1 -> Gain64/1
  Integrator34/1 -> Display10/1
  Derivative12/1 -> Product20/2
  Sum117/1 -> Wind12/1
  First Order Hold94/1 -> Sum154/1
  Integrator31/1 -> Manual Variant Source26/1, Product18/1
  Uniform Random Number61/1 -> First Order Hold87/1
  Integrator33/1 -> Manual Variant Source24/2, Product23/2
  Sum138/1 -> Sum134/2
  Transfer Fcn59/1 -> Sum118/1
  Sum120/1 -> Sum141/2
  Manual Variant Source26/1 -> Manual Variant Source19/1
  Uniform Random Number56/1 -> First Order Hold75/1
  Transfer Fcn54/1 -> GRC10/1
  First Order Hold92/1 -> Sum155/1
  Sum147/1 -> Sum139/1
  Manual Variant Source24/1 -> Manual Variant Source27/1
  Uniform Random Number64/1 -> First Order Hold91/1
  Integrator35/1 -> Display11/1
  Sum119/1 -> Solar12/1
  First Order Hold78/1 -> Sum126/1
  Constant5/1 -> MPC Controller2/2
  Constant3/1 -> MPC Controller1/2
  Transfer Fcn56/1 -> Gain54/1, Derivative12/1, MPC Controller/1, PowerPlant7/1, Abs9/1, Sum151/1, Transfer Fcn47/1, Gain50/1, Gain60/1
  Constant4/1 -> MPC Controller/2
  Transfer Fcn42/1 -> Gain44/1, PID Controller1/1, Derivative7/1, Transfer Fcn44/1, Sum96/1, Frequency/4, Abs7/1, Gain38/1, Gain25/1
  Transfer Fcn43/1 -> Frequency/6, Abs8/1, Sum97/1, Transfer Fcn33/1, Gain45/1, Gain42/1, Derivative8/1, PID Controller3/1, Gain39/1
  Sum145/1 -> Sum144/2, MPC Controller/3, PowerPlant6/3
  Transfer Fcn28/1 -> To Workspace17/1, Frequency/5, Abs5/1, Sum58/1, Transfer Fcn18/1, Gain33/1, Gain30/1, Derivative5/1, Gain24/1, Mux3/1
  Transfer Fcn27/1 -> Gain32/1, Derivative4/1, Mux2/1, Transfer Fcn29/1, Sum57/1, Gain18/1, To Workspace16/1, Frequency/3, Abs4/1, Gain23/1
  Transfer Fcn26/1 -> Gain22/1, Mux1/1, Derivative6/1, To Workspace15/1, Frequency/1, Abs3/1, Sum56/1, Transfer Fcn17/1, Gain19/1, Gain31/1
